simulink model "exp8_6"  (R2023a)
settings: Solver=VariableStepAuto  StartTime=0.0  StopTime=10.0  RelTol=1e-3
libraries: dspfdesign x1
settings Model: Creator=Lenovo  LastModifiedBy=Lenovo

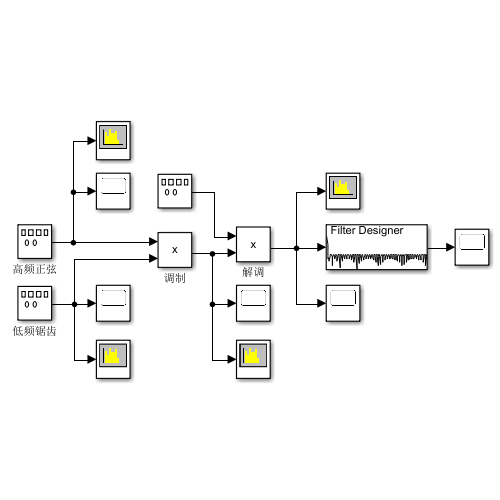
[thumbnail: Simulink's stored preview of the top-level diagram]
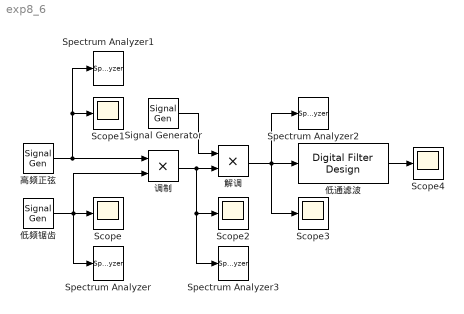
== system exp8_6 ==
  Scope{,1..4} (5 alike) : Scope
  Signal Generator : SignalGenerator  Frequency=50*pi  Units=rad/sec
  Spectrum Analyzer : SpectrumAnalyzer  WindowPosition=[700.000000,181.000000,800.000000,500.000000,]  ScopeFrameLocation=window  YLimits=[-53.90048817,31.90113197]  ColorLimits=[-80 20]
  Spectrum Analyzer1 : SpectrumAnalyzer  WindowPosition=[571.000000,756.000000,800.000000,500.000000,]  ScopeFrameLocation=window  YLimits=[-148.33940579,39.99266406]  ColorLimits=[-80 20]
  Spectrum Analyzer2 : SpectrumAnalyzer  WindowPosition=[1421.000000,734.000000,800.000000,500.000000,]  ScopeFrameLocation=window  YLimits=[-211.81638849,42.76231994]  ColorLimits=[-80 20]
  Spectrum Analyzer3 : SpectrumAnalyzer  WindowPosition=[700.000000,181.000000,800.000000,500.000000,]  ScopeFrameLocation=window  YLimits=[-92.21551396,25.81379883]  ColorLimits=[-80 20]
  低通滤波 : dspfdesign/Digital Filter Design  mwdsp_browser_bugfix_var=off
  低频锯齿 : SignalGenerator  WaveForm=sawtooth  Frequency=pi  Units=rad/sec
  解调 : Product
  调制 : Product
  高频正弦 : SignalGenerator  Frequency=50*pi  Units=rad/sec
  wires:
  高频正弦/1 -> Spectrum Analyzer1/1, Scope1/1, 调制/1
  低频锯齿/1 -> 调制/2, Spectrum Analyzer/1, Scope/1
  调制/1 -> Spectrum Analyzer3/1, Scope2/1, 解调/2
  Signal Generator/1 -> 解调/1
  解调/1 -> Scope3/1, 低通滤波/1, Spectrum Analyzer2/1
  低通滤波/1 -> Scope4/1
